simulink model "dof2_Arm"  (R2025a)
settings: Solver=VariableStepAuto  StartTime=0.0  StopTime=30  RelTol=1e-3
PreLoadFcn:
  | A = [0 0 1.000000000000000 0;
  |      0 0 0 1.000000000000000;
  |      11.559078600576106 11.559058468503522 0 0;
  |      -57.472982345831987 -57.472932960268153 0 0];
  | 
  | B = [0 0;
  |      0 0;
  |      10.7031392416673 -26.2556457650549;
  |      -26.2556457650549 103.5844495961264];
  | 
  | C = [1 0 0 0;
  |      0 1 0 0];
  | 
  | D = [0 0;
  |      0 0];
StopFcn:
  | Xd = Desired.Data(:,1);
  | Yd = Desired.Data(:,2);
  | Xa = Actual.Data(:,1);
  | Ya = Actual.Data(:,2);
  | 
  | % v = VideoWriter('introducing_disturbance.avi');
  | % v.FrameRate = 30; % You may lower this if desired
  | % open(v);
  | 
  | figure;
  | subplot(1,2,1);
  | h1 = animatedline('Color','r','LineWidth',2);
  | title('Desired Trajectory');
  | xlabel('X'); ylabel('Y'); axis equal; grid on;
  | xlim([min([Xd;Xa])-0.5, max([Xd;Xa])+0.5]);
  | ylim([min([Yd;Ya])-0.5, max([Yd;Ya])+0.5]);
  | 
  | subplot(1,2,2);
  | h2 = animatedline('Color','b','LineWidth',2);
  | title('Actual Trajectory');
  | xlabel('X'); ylabel('Y'); axis equal; grid on;
  | xlim([min([Xd;Xa])-0.5, max([Xd;Xa])+0.5]);
  | ylim([min([Yd;Ya])-0.5, max([Yd;Ya])+0.5]);
  | 
  | N = min(length(Xd), length(Xa));
  | skip = 10; % Record every 10th sample for faster video
  | 
  | for k = 1:skip:N
  |     addpoints(h1, Xd(k), Yd(k));
  |     addpoints(h2, Xa(k), Ya(k));
  |     drawnow;
  |     % frame = getframe(gcf);
  |     % writeVideo(v, frame);
  | end
  | 
  | % close(v);
  | % disp('Animation saved');
libraries: slpidlib x2
settings Model: Creator=LENOVO  LastModifiedBy=LENOVO
settings DataIOCC: SaveOutput=off  SaveTime=off  ReturnWorkspaceOutputs=off
settings DebuggingCC: AlgebraicLoopMsg=none
settings ExplorerConfigSet: InternalSimMechanicsExplorerSettings=|
  | <ExplorerConfiguration>
  | 
  |   <canonicalview>default</canonicalview>
  | 
  |   <TilePanel>
  |     <TileInfo>
  |       <Tiles Columns="1" Count="1" Height="608" Rows="1" Width="1079">
  |         <Row Weight="1"/>
  |         <Column Weight="1"/>
  |         <Tile Height="1" Width="1" X="0" Y="0"/>
  |       </Tiles>
  |     </TileInfo>
  |     <SceneInfo>
  |       <SceneViewer>
  |         <IsThisViewStd>
  |           <IsStandardView>off</IsStandardView>
  |           <StandardViewName>Front</StandardViewName>
  |         </IsThisViewStd>
  |         <BGColor>
  |           <R>1</R>
  |           <G>1</G>
  |           <B>1</B>
  |           <A>1</A>
  |         </BGColor>
  |         <Camera>
  |           <DoPerspective>off</DoPerspective>
  |           <Position>
  |             <X>1.2314400000000001</X>
  |             <Y>-1.05352</Y>
  |             <Z>-0.27438000000000001</Z>
  |           </Position>
  |           <Center>
  |             <X>0.17921000000000001</X>
  |             <Y>-0.0012899999999999999</Y>
  |             <Z>-0.27438000000000001</Z>
  |           </Center>
  |           <Up>
  |             <X>0</X>
  |             <Y>0</Y>
  |             <Z>1</Z>
  |           </Up>
  |           <XLim>1.0678484236679733</XLim>
  |           <YLim>1.0678484236679733</YLim>
  |           <ViewLimDist>0.01</ViewLimDist>
  |         </Camera>
  |       </SceneViewer>
  |     </SceneInfo>
  |   </TilePanel>
  | 
  |   <MechEditorPanel>
  |     <GfxPanelCameraMap/>
  |     <Cameras/>
  |     <VideoCreator>
  |       <IncludeTiles>All</IncludeTiles>
  |       <IncludeTime>on</IncludeTime>
  |       <IncludeWorldFrame>off</IncludeWorldFrame>
  |       <PlaybackSpeedRatio>1</PlaybackSpeedRatio>
  |       <FrameRate>30</FrameRate>
  |       <FrameSize>auto</FrameSize>
  |       <VideoFormat>UncompressedAVI</VideoFormat>
  |     </VideoCreator>
  |   </MechEditorPanel>
  | 
  |   <PlaybackSettings>
  |     <PlaybackSpeedFactor>8</PlaybackSpeedFactor>
  |   </PlaybackSettings>
  | 
  | </ExplorerConfiguration>

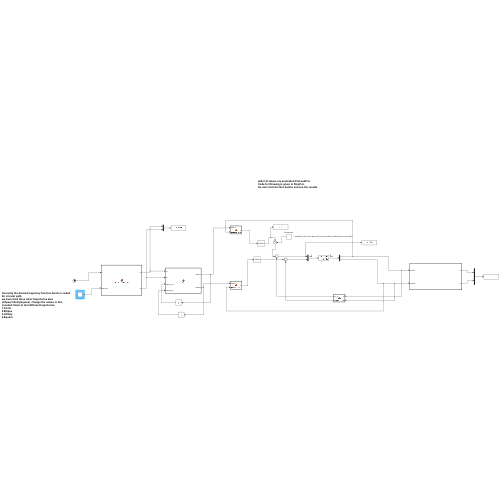
[thumbnail: Simulink's stored preview of the top-level diagram]
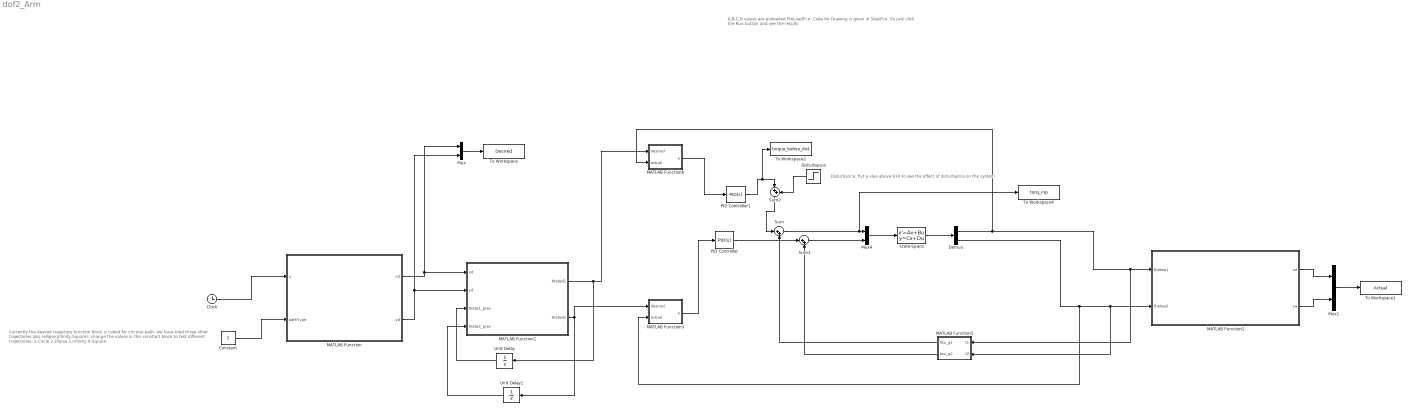
== system dof2_Arm ==
  note: Disturbance. Put a vlue above 830 to see the affect of disturbance on the system
  note: Currently the desired trajectory function block is coded for circular path.
      | we have tried three other trajectories also (ellipse,infinity,Square). change the values in this constant block to test different trajectories.
      | 1.Circle
      | 2.Ellipse
      | 3.Infinity
      | 4.Square
  note: A,B,C,D values are preloaded PreLoadFcn.
      | Code for Drawing is given in StopFcn.
      | So Just click the Run button and see the results
  Clock : Clock
  Constant : Constant
  Demux : Demux  Outputs=2
  Disturbance : Step  Time=10  After=1000  SampleTime=0
  MATLAB Function : MATLAB Function  TreatAsAtomicUnit=on
  MATLAB Function1 : MATLAB Function  TreatAsAtomicUnit=on
  MATLAB Function2 : MATLAB Function  TreatAsAtomicUnit=on
  MATLAB Function3 : MATLAB Function  TreatAsAtomicUnit=on
  MATLAB Function5 : MATLAB Function  TreatAsAtomicUnit=on
  MATLAB Function6 : MATLAB Function  TreatAsAtomicUnit=on
  Mux : Mux  Inputs=2
  Mux1 : Mux  Inputs=2
  Mux4 : Mux  Inputs=2
  PID Controller : slpidlib/PID Controller  Controller=PID  Form=Parallel  TimeDomain=Continuous-time  UseExternalTs=off  SampleTime=-1  IntegratorMethod=Forward Euler  FilterMethod=Forward Euler  ControllerParametersSource=internal  P=6376.05236292116  I=588535.84447394  UseKiTs=off  D=17.0517552352624  UseExternalDerivativeSource=off  N=19173.6461685568  UseFilter=on  TunerSelectOption=Transfer Function Based (PID Tuner App)  InitialConditionSource=internal  InitialConditionForIntegrator=0  InitialConditionForFilter=0  DifferentiatorICPrevScaledInput=0  ExternalReset=none  TrackingMode=off  Kt=1  LimitOutput=off  SatLimitsSource=internal  UpperSaturationLimit=inf  LowerSaturationLimit=-inf  LinearizeAsGain=on  AntiWindupMode=none  Kb=1  LimitIntegrator=off  UpperIntegratorSaturationLimit=inf  LowerIntegratorSaturationLimit=-inf  POutMin=[]  POutMax=[]  IOutMin=[]  IOutMax=[]  DOutMin=[]  DOutMax=[]  NOutMin=[]  NOutMax=[]  SumOutMin=[]  SumOutMax=[]  SaturationOutMin=[]  SaturationOutMax=[]  PParamMin=[]  PParamMax=[]  IParamMin=[]  IParamMax=[]  DParamMin=[]  DParamMax=[]  NParamMin=[]  NParamMax=[]  KbParamMin=[]  KbParamMax=[]  KtParamMin=[]  KtParamMax=[]  KbOutMin=[]  KbOutMax=[]  KtOutMin=[]  KtOutMax=[]  IntegratorOutMin=[]  IntegratorOutMax=[]  FilterOutMin=[]  FilterOutMax=[]  SumI1OutMin=[]  SumI1OutMax=[]  SumI2OutMin=[]  SumI2OutMax=[]  SumI3OutMin=[]  SumI3OutMax=[]  SumI4OutMin=[]  SumI4OutMax=[]  SumDOutMin=[]  SumDOutMax=[]  DifferentiatorOutMin=[]  DifferentiatorOutMax=[]  FilterDiffOutCoefMin=[]  FilterDiffOutCoefMax=[]  ReciprocalOutMin=[]  ReciprocalOutMax=[]  SumDenOutMin=[]  SumDenOutMax=[]  SumNumOutMin=[]  SumNumOutMax=[]  DivideOutMin=[]  DivideOutMax=[]  UdiffTsProdOutMin=[]  UdiffTsProdOutMax=[]  NTsProdOutMin=[]  NTsProdOutMax=[]  UintegralTsProdOutMin=[]  UintegralTsProdOutMax=[]  UngainTsProdOutMin=[]  UngainTsProdOutMax=[]  ClampingZeroOutDataTypeStr=Inherit: Inherit via back propagation  ClampingZeroOutMin=[]  ClampingZeroOutMax=[]  FilterDenConstantOutDataTypeStr=Inherit: Inherit via back propagation  FilterDenConstantOutMin=[]  FilterDenConstantOutMax=[]  PCopyOutDataTypeStr=Inherit: Inherit via back propagation  PCopyOutMin=[]  PCopyOutMax=[]  NCopyOutDataTypeStr=Inherit: Inherit via back propagation  NCopyOutMin=[]  NCopyOutMax=[]  IntegratorContinuousStateAttributes=''  IntegratorStateMustResolveToSignalObject=off  IntegratorRTWStateStorageClass=Auto  FilterContinuousStateAttributes=''  FilterStateMustResolveToSignalObject=off  FilterRTWStateStorageClass=Auto  ParallelPVariant=InternalParameters  IdealPVariant=Disabled  IVariant=InternalParameters  DVariant=InternalParameters  IntegratorVariant=Continuous  SatVariant=Disabled  AWVariant=Passthrough  PCopyVariant=Disabled  TRVariant=Disabled  FdbkBlocksVariant=Forward  IdealPFdbkVariant=Disabled  SatFdbkVariant=Disabled  DerivativeFilterVariant=ContFilter  NVariant=InternalParameters  NCopyVariant=Disabled  FilterICVariant=InternalICsFilter  IntegratorICVariant=InternalICs  ExternalResetVariant=Disabled  TRSumVariant=Passthrough  SumFdbkVariant=Disabled  SumVariant=Sum_PID  TsampFilterVariant=InternalTs  TsampNgainVariant=Passthrough  TsampIntegralVariant=Disabled_SignalSpec  ExternalSaturationOutDataTypeStr=Inherit: Same as second input  DerivativeSourceVariant=ErrorSignal  PreIntVariant=InternalPreInt
  PID Controller1 : slpidlib/PID Controller  Controller=PID  Form=Parallel  TimeDomain=Continuous-time  UseExternalTs=off  SampleTime=-1  IntegratorMethod=Forward Euler  FilterMethod=Forward Euler  ControllerParametersSource=internal  P=238.450973556947  I=155.241483890582  UseKiTs=off  D=21.1635823866133  UseExternalDerivativeSource=off  N=9060.93075425275  UseFilter=on  TunerSelectOption=Transfer Function Based (PID Tuner App)  InitialConditionSource=internal  InitialConditionForIntegrator=0  InitialConditionForFilter=0  DifferentiatorICPrevScaledInput=0  ExternalReset=none  TrackingMode=off  Kt=1  LimitOutput=off  SatLimitsSource=internal  UpperSaturationLimit=inf  LowerSaturationLimit=-inf  LinearizeAsGain=on  AntiWindupMode=none  Kb=1  LimitIntegrator=off  UpperIntegratorSaturationLimit=inf  LowerIntegratorSaturationLimit=-inf  POutMin=[]  POutMax=[]  IOutMin=[]  IOutMax=[]  DOutMin=[]  DOutMax=[]  NOutMin=[]  NOutMax=[]  SumOutMin=[]  SumOutMax=[]  SaturationOutMin=[]  SaturationOutMax=[]  PParamMin=[]  PParamMax=[]  IParamMin=[]  IParamMax=[]  DParamMin=[]  DParamMax=[]  NParamMin=[]  NParamMax=[]  KbParamMin=[]  KbParamMax=[]  KtParamMin=[]  KtParamMax=[]  KbOutMin=[]  KbOutMax=[]  KtOutMin=[]  KtOutMax=[]  IntegratorOutMin=[]  IntegratorOutMax=[]  FilterOutMin=[]  FilterOutMax=[]  SumI1OutMin=[]  SumI1OutMax=[]  SumI2OutMin=[]  SumI2OutMax=[]  SumI3OutMin=[]  SumI3OutMax=[]  SumI4OutMin=[]  SumI4OutMax=[]  SumDOutMin=[]  SumDOutMax=[]  DifferentiatorOutMin=[]  DifferentiatorOutMax=[]  FilterDiffOutCoefMin=[]  FilterDiffOutCoefMax=[]  ReciprocalOutMin=[]  ReciprocalOutMax=[]  SumDenOutMin=[]  SumDenOutMax=[]  SumNumOutMin=[]  SumNumOutMax=[]  DivideOutMin=[]  DivideOutMax=[]  UdiffTsProdOutMin=[]  UdiffTsProdOutMax=[]  NTsProdOutMin=[]  NTsProdOutMax=[]  UintegralTsProdOutMin=[]  UintegralTsProdOutMax=[]  UngainTsProdOutMin=[]  UngainTsProdOutMax=[]  ClampingZeroOutDataTypeStr=Inherit: Inherit via back propagation  ClampingZeroOutMin=[]  ClampingZeroOutMax=[]  FilterDenConstantOutDataTypeStr=Inherit: Inherit via back propagation  FilterDenConstantOutMin=[]  FilterDenConstantOutMax=[]  PCopyOutDataTypeStr=Inherit: Inherit via back propagation  PCopyOutMin=[]  PCopyOutMax=[]  NCopyOutDataTypeStr=Inherit: Inherit via back propagation  NCopyOutMin=[]  NCopyOutMax=[]  IntegratorContinuousStateAttributes=''  IntegratorStateMustResolveToSignalObject=off  IntegratorRTWStateStorageClass=Auto  FilterContinuousStateAttributes=''  FilterStateMustResolveToSignalObject=off  FilterRTWStateStorageClass=Auto  ParallelPVariant=InternalParameters  IdealPVariant=Disabled  IVariant=InternalParameters  DVariant=InternalParameters  IntegratorVariant=Continuous  SatVariant=Disabled  AWVariant=Passthrough  PCopyVariant=Disabled  TRVariant=Disabled  FdbkBlocksVariant=Forward  IdealPFdbkVariant=Disabled  SatFdbkVariant=Disabled  DerivativeFilterVariant=ContFilter  NVariant=InternalParameters  NCopyVariant=Disabled  FilterICVariant=InternalICsFilter  IntegratorICVariant=InternalICs  ExternalResetVariant=Disabled  TRSumVariant=Passthrough  SumFdbkVariant=Disabled  SumVariant=Sum_PID  TsampFilterVariant=InternalTs  TsampNgainVariant=Passthrough  TsampIntegralVariant=Disabled_SignalSpec  ExternalSaturationOutDataTypeStr=Inherit: Same as second input  DerivativeSourceVariant=ErrorSignal  PreIntVariant=InternalPreInt
  State-Space : StateSpace  A=A  B=B  C=C  D=D  InitialCondition=0
  Sum : Sum  Inputs=|++
  Sum1 : Sum  Inputs=|++
  Sum2 : Sum  Inputs=|++
  To Workspace : ToWorkspace  VariableName=Desired  SaveFormat=Timeseries  SampleTime=-1
  To Workspace1 : ToWorkspace  VariableName=Actual  SaveFormat=Timeseries  SampleTime=-1
  To Workspace2 : ToWorkspace  VariableName=torque_before_dist  SaveFormat=Timeseries  SampleTime=-1
  To Workspace4 : ToWorkspace  VariableName=torq_inp  SaveFormat=Timeseries  SampleTime=-1
  Unit Delay : UnitDelay  SampleTime=-1  HasFrameUpgradeWarning=on
  Unit Delay1 : UnitDelay  SampleTime=-1  HasFrameUpgradeWarning=on
  wires:
  Clock/1 -> MATLAB Function/1(u)
  MATLAB Function/1(xd) -> Mux/1, MATLAB Function1/1(xd)
  MATLAB Function/2(yd) -> Mux/2, MATLAB Function1/2(yd)
  MATLAB Function2/2(ya) -> Mux1/2
  MATLAB Function2/1(xa) -> Mux1/1
  Mux/1 -> To Workspace/1
  Mux1/1 -> To Workspace1/1
  MATLAB Function1/2(thetad2) -> Unit Delay1/1, MATLAB Function3/1(desired)
  Unit Delay/1 -> MATLAB Function1/3(theta1_prev)
  Unit Delay1/1 -> MATLAB Function1/4(theta2_prev)
  MATLAB Function6/1(e) -> PID Controller1/1
  MATLAB Function3/1(e) -> PID Controller/1
  MATLAB Function5/1(tau_g1) -> Sum/2
  PID Controller/1 -> Sum1/1
  MATLAB Function5/2(tau_g2) -> Sum1/2
  Demux/1 -> MATLAB Function2/1(thetaa1), MATLAB Function5/1(t1), MATLAB Function6/2(actual)
  Demux/2 -> MATLAB Function2/2(thetaa2), MATLAB Function5/2(t2), MATLAB Function3/2(actual)
  Mux4/1 -> State-Space/1
  MATLAB Function1/1(thetad1) -> Unit Delay/1, MATLAB Function6/1(desired)
  Sum1/1 -> Mux4/2
  State-Space/1 -> Demux/1
  PID Controller1/1 -> To Workspace2/1, Sum2/1
  Sum/1 -> To Workspace4/1, Mux4/1
  Disturbance/1 -> Sum2/2
  Sum2/1 -> Sum/1
  Constant/1 -> MATLAB Function/2(pathType)

== matlab function dof2_Arm/MATLAB Function1 ==
  data: thetad1 output; thetad2 output; xd input; yd input; theta1_prev input; theta2_prev input
function [thetad1,thetad2] = inverse_kinematics(xd, yd, theta1_prev, theta2_prev)
l1 = 0.3;
l2 = 0.25;
cos_t2 = (xd^2 + yd^2 - l1^2 - l2^2) / (2*l1*l2);
cos_t2 = max(min(cos_t2, 1), -1);  
sin_t2_1 =  sqrt(1 - cos_t2^2);  % Elbow-down solution
sin_t2_2 = -sqrt(1 - cos_t2^2);  % Elbow-up solution

% Two possible theta2 values
theta2_1 = atan2(sin_t2_1, cos_t2);
theta2_2 = atan2(sin_t2_2, cos_t2);

% Compute corresponding theta1 for each solution
k1 = l1 + l2*cos_t2;
k2_1 = l2*sin_t2_1;
k2_2 = l2*sin_t2_2;
theta1_1 = atan2(yd, xd) - atan2(k2_1, k1); % Elbow-down
theta1_2 = atan2(yd, xd) - atan2(k2_2, k1); % Elbow-up

candidates = [theta1_1, theta2_1; theta1_2, theta2_2];

% If previous joint angles provided, select solution with minimal difference
if nargin == 4
    diffs = sum(abs(candidates - [theta1_prev, theta2_prev]), 2);
    [~, idx] = min(diffs);
else
    idx = 1; % Default: Elbow-down
end

thetad1 = candidates(idx, 1);
thetad2 = candidates(idx, 2);
end

== matlab function dof2_Arm/MATLAB Function ==
  data: u input; xd output; yd output; pathType input
function [xd, yd] = Desired_Trajectory(u, pathType)
% pathType: 1 = circle, 2 = ellipse, 3 = figure8, 4 = square

    switch pathType
        case 1 % Circle
            r = 0.5;
            theta = (2*pi/6)*u;
            xc = 0; yc = 0;
            xd = xc + r*cos(theta);
            yd = yc + r*sin(theta);

        case 2 % Ellipse
            a = 0.45; b = 0.25;
            theta = (2*pi/6)*u;
            xc = 0; yc = 0;
            xd = xc + a*cos(theta);
            yd = yc + b*sin(theta);

        case 3 % Figure 8
            a = 0.25;
            theta = (2*pi/6)*u;
            xc = 0; yc = 0;
            xd = xc + a*sin(theta);
            yd = yc + a*sin(theta).*cos(theta);

        case 4 % Square
            r = 0.35;
            xc = 0; yc = 0;
            theta = mod(u,4);
            if theta < 1
                xd = xc + r;
                yd = yc + r * (theta);
            elseif theta < 2
                xd = xc + r - r * (theta-1);
                yd = yc + r;
            elseif theta < 3
                xd = xc - r;
                yd = yc + r - r * (theta-2);
            else
                xd = xc - r + r * (theta-3);
                yd = yc - r;
            end

        otherwise
            xd = 0;
            yd = 0;
    end
end

== matlab function dof2_Arm/MATLAB Function2 ==
  data: xa output; ya output; thetaa1 input; thetaa2 input
function [xa,ya] = Forward_Kinematics(thetaa1,thetaa2)
l1=0.3;
l2=0.25;
xa=l1*cos(thetaa1)+l2*cos(thetaa1+thetaa2);
ya=l1*sin(thetaa1)+l2*sin(thetaa1+thetaa2);

== matlab function dof2_Arm/MATLAB Function3 ==
  data: desired input; actual input; e output
function e = wrapped_error(desired,actual)
e = atan2(sin(desired - actual), cos(desired - actual));
end

== matlab function dof2_Arm/MATLAB Function5 ==
  data: t1 input; tau_g1 output; t2 input; tau_g2 output
function [tau_g1, tau_g2] = gravity_comp(t1, t2)

m1 = 1.37;
m2 = 1.16;
l1 = 0.3;
lc1 = 0.15;
lc2 = 0.125;
g = 9.81;

tau_g1 = (m1*lc1 + m2*l1)*g*cos(t1) + m2*lc2*g*cos(t1 + t2);
tau_g2 = m2*lc2*g*cos(t1 + t2);
end

== matlab function dof2_Arm/MATLAB Function6 ==
  data: desired input; actual input; e output
function e = wrapped_error(desired,actual)
e = atan2(sin(desired - actual), cos(desired - actual));
end
